simulink model "invarianza_temporal"  (R2018a)
settings: Solver=VariableStepAuto  StartTime=0.0  StopTime=20  MaxStep=1e-2  RelTol=1e-3
settings Model: Creator=carma  LastModifiedBy=carma

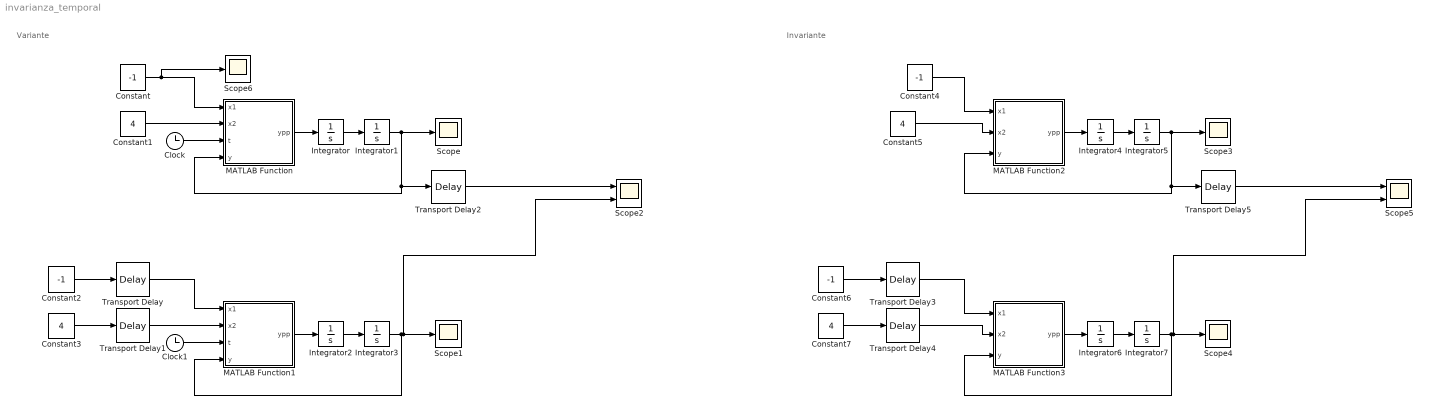
== system invarianza_temporal ==
  note: Variante
  note: Invariante
  Clock : Clock
  Clock1 : Clock
  Constant{,2,4,6} (4 alike) : Constant  Value=-1
  Constant{1,3,5,7} (4 alike) : Constant  Value=4
  Integrator{,1..7} (8 alike) : Integrator
  MATLAB Function : MATLAB Function  TreatAsAtomicUnit=on
  MATLAB Function1 : MATLAB Function  TreatAsAtomicUnit=on
  MATLAB Function2 : MATLAB Function  TreatAsAtomicUnit=on
  MATLAB Function3 : MATLAB Function  TreatAsAtomicUnit=on
  Scope{,1,3..4,6} (5 alike) : Scope
  Scope2 : Scope  NumInputPorts=2
  Scope5 : Scope  NumInputPorts=2
  Transport Delay{,1..5} (6 alike) : TransportDelay  DelayTime=3
  wires:
  Constant/1 -> Scope6/1, MATLAB Function/1(x1)
  Constant1/1 -> MATLAB Function/2(x2)
  Clock/1 -> MATLAB Function/3(t)
  MATLAB Function/1(ypp) -> Integrator/1
  Integrator/1 -> Integrator1/1
  Clock1/1 -> MATLAB Function1/3(t)
  Constant2/1 -> Transport Delay/1
  Constant3/1 -> Transport Delay1/1
  Integrator3/1 -> Scope2/2, Scope1/1, MATLAB Function1/4(y)
  MATLAB Function1/1(ypp) -> Integrator2/1
  Integrator2/1 -> Integrator3/1
  Transport Delay/1 -> MATLAB Function1/1(x1)
  Transport Delay1/1 -> MATLAB Function1/2(x2)
  Integrator1/1 -> Scope/1, MATLAB Function/4(y), Transport Delay2/1
  Transport Delay2/1 -> Scope2/1
  Integrator6/1 -> Integrator7/1
  Constant7/1 -> Transport Delay4/1
  MATLAB Function3/1(ypp) -> Integrator6/1
  Constant6/1 -> Transport Delay3/1
  Transport Delay5/1 -> Scope5/1
  Transport Delay4/1 -> MATLAB Function3/2(x2)
  Integrator7/1 -> Scope5/2, Scope4/1, MATLAB Function3/3(y)
  Transport Delay3/1 -> MATLAB Function3/1(x1)
  Constant4/1 -> MATLAB Function2/1(x1)
  Constant5/1 -> MATLAB Function2/2(x2)
  Integrator5/1 -> Scope3/1, Transport Delay5/1, MATLAB Function2/3(y)
  MATLAB Function2/1(ypp) -> Integrator4/1
  Integrator4/1 -> Integrator5/1

== matlab function invarianza_temporal/MATLAB Function1 ==
  data: x1 input; ypp output; x2 input; t input; y input
function ypp = fcn(x1,x2,t,y)

ypp=(5*cos(t)*x1+4*x2-5*exp(t)*y)/3;

== matlab function invarianza_temporal/MATLAB Function ==
  data: x1 input; ypp output; x2 input; t input; y input
function ypp = fcn(x1,x2,t,y)

ypp=(5*cos(t)*x1+4*x2-5*exp(t)*y)/3;

== matlab function invarianza_temporal/MATLAB Function2 ==
  data: x1 input; ypp output; x2 input; y input
function ypp = fcn(x1,x2,y)

ypp=(5*x1+4*x2-5*y)/3;

== matlab function invarianza_temporal/MATLAB Function3 ==
  data: x1 input; ypp output; x2 input; y input
function ypp = fcn(x1,x2,y)

ypp=(5*x1+4*x2-5*y)/3;
